simulink model "flatball_6dof-old"  (R2021b)
settings: Solver=ode1be  StartTime=0.0  StopTime=10  FixedStep=0.001  MaxStep=0.01  MinStep=0.01  RelTol=1e-3
values from neighbouring files (symbols this model uses):
  amb = evalin( 'base', 'amb')    [flatball_6dof_eqom.m]
  disc = evalin( 'base', 'disc')    [flatball_6dof_eqom.m]    (also in flatball_6dof_init.m = struct; flatball_init_disc_params.m = struct)
libraries: matrix_library x2, aerolibanim x1, simulink x1
(part 1 of 2)
settings Model: Creator=schae  LastModifiedBy=schae
settings SolverCC: InitialStep=0.01
settings DataIOCC: ReturnWorkspaceOutputsName=simout

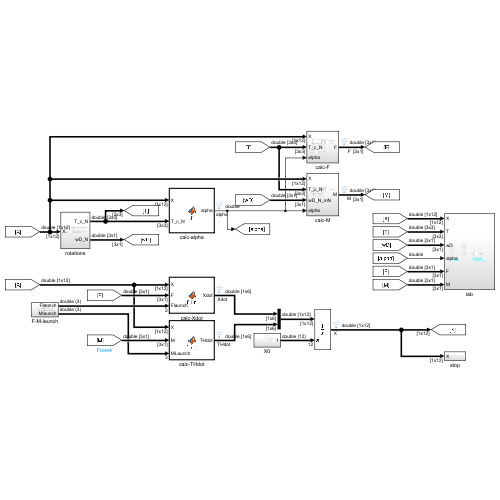
[thumbnail: Simulink's stored preview of the top-level diagram]
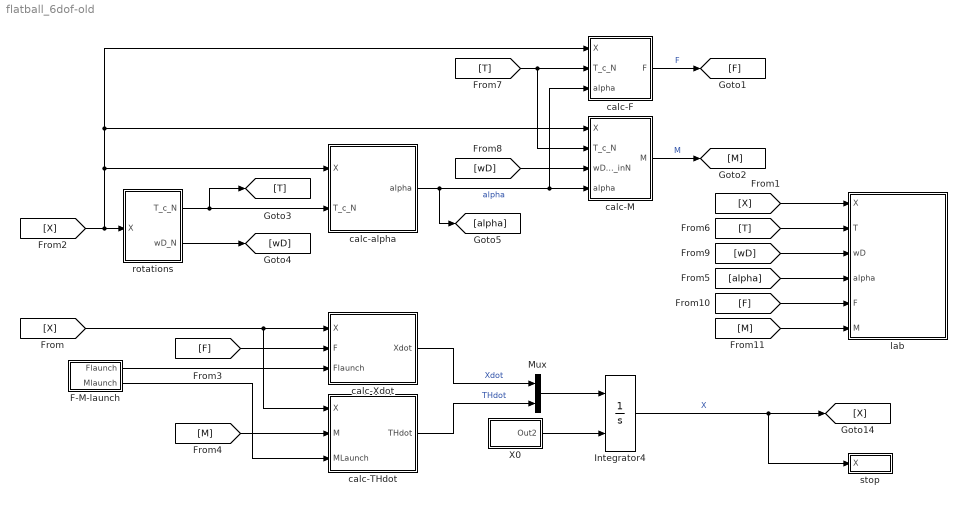
== system flatball_6dof-old ==
  F-M-launch : Subsystem
  Integrator4 : Integrator  InitialConditionSource=external
  Mux : Mux  Inputs=2
  X0 : Subsystem
  calc-F : Subsystem
  calc-M : Subsystem
  calc-THdot : MATLAB Function  TreatAsAtomicUnit=on
  calc-Xdot : MATLAB Function  TreatAsAtomicUnit=on
  calc-alpha : MATLAB Function  TreatAsAtomicUnit=on
  lab : Subsystem
  rotations : Subsystem
  stop : Subsystem
  wires:
  calc-Xdot/1(Xdot) -> Mux/1  "Xdot"
  X0/1(Out2) -> Integrator4/2
  Integrator4/1 -> stop/1(X), [X]  "X"
  [X] -> calc-THdot/1(X), calc-Xdot/1(X)
  calc-THdot/1(THdot) -> Mux/2  "THdot"
  Mux/1 -> Integrator4/1
  [wD] -> calc-M/3(wD_N_inN)
  calc-alpha/1(alpha) -> [alpha], calc-F/3(alpha), calc-M/4(alpha)  "alpha"
  rotations/1(T_c_N) -> [T], calc-alpha/2(T_c_N)
  rotations/2(wD_N) -> [wD]
  calc-F/1(F) -> [F]  "F"
  calc-M/1(M) -> [M]  "M"
  [T] -> calc-M/2(T_c_N), calc-F/2(T_c_N)
  [X] -> calc-F/1(X), calc-M/1(X), calc-alpha/1(X), rotations/1(X)
  [X] -> lab/1(X)
  [M] -> calc-THdot/2(M)
  [F] -> calc-Xdot/2(F)
  [T] -> lab/2(T)
  [wD] -> lab/3(wD)
  [F] -> lab/5(F)
  [M] -> lab/6(M)
  [alpha] -> lab/4(alpha)
  F-M-launch/1(Flaunch) -> calc-Xdot/3(Flaunch)
  F-M-launch/2(Mlaunch) -> calc-THdot/3(MLaunch)

== system flatball_6dof-old/F-M-launch ==
  Scope : Scope  NumInputPorts=2
  Subsystem : Subsystem
  Subsystem1 : Subsystem
  X0_hummel_f2302 : Constant  Commented=on  Value=[-0.90 -0.63 -0.91 13.42 -0.41 0.001 -0.07 0.21 5.03 -14.94 -1.48 54.25]
  Flaunch : Outport
  Mlaunch : Outport  Port=2
  wires:
  Subsystem1/1(Mlaunch) -> Scope/2, Mlaunch/1
  Subsystem/1(Flaunch) -> Scope/1, Flaunch/1

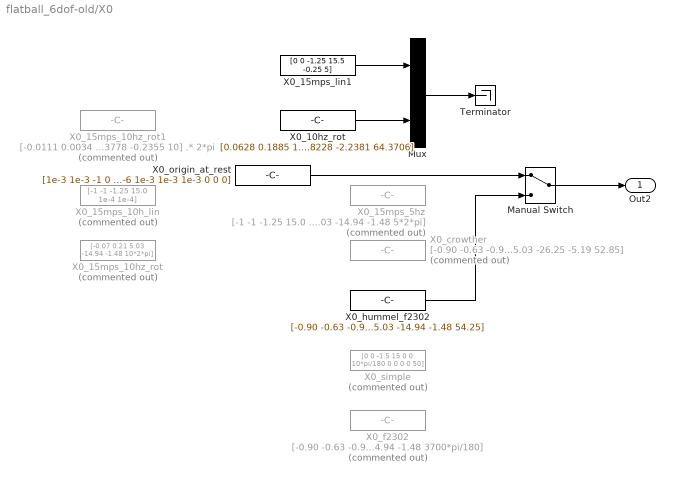
== system flatball_6dof-old/X0 ==
  Manual Switch : ManualSwitch
  Mux : Mux  Inputs=2
  Terminator : Terminator
  X0_10hz_rot : Constant  Value=[0.0628 0.1885 12.5664 1.8228 -2.2381 64.3706]
  X0_15mps_10h_lin : Constant  Commented=on  Value=[-1 -1 -1.25 15.0 1e-4 1e-4]
  X0_15mps_10hz_rot : Constant  Commented=on  Value=[-0.07 0.21 5.03 -14.94 -1.48 10*2*pi]
  X0_15mps_10hz_rot1 : Constant  Commented=on  Value=[-0.0111 0.0034 0.8005 -2.3778 -0.2355 10] .* 2*pi
  X0_15mps_5hz : Constant  Commented=on  Value=[-1 -1 -1.25 15.0 1e-4 1e-4 -0.07 0.21 5.03 -14.94 -1.48 5*2*pi]
  X0_15mps_lin1 : Constant  Value=[0 0 -1.25 15.5 -0.25 5]
  X0_crowther : Constant  Commented=on  Value=[-0.90 -0.63 -0.91 4.48 12.52 1.84 -0.07 0.21 5.03 -26.25 -5.19 52.85]
  X0_f2302 : Constant  Commented=on  Value=[-0.90 -0.63 -0.91 13.42 -0.41 0.001 -0.07 0.21 5.03 -14.94 -1.48 3700*pi/180]
  X0_hummel_f2302 : Constant  Value=[-0.90 -0.63 -0.91 13.42 -0.41 0.001 -0.07 0.21 5.03 -14.94 -1.48 54.25]
  X0_origin_at_rest : Constant  Value=[1e-3 1e-3 -1 0 0 -1e-6 1e-3 1e-3 1e-3 0 0 0]
  X0_simple : Constant  Commented=on  Value=[0 0 -1.5 15 0 0 10*pi/180 0 0 0 0 50]
  Out2 : Outport
  wires:
  Manual Switch/1 -> Out2/1
  X0_10hz_rot/1 -> Mux/2
  X0_15mps_lin1/1 -> Mux/1
  X0_hummel_f2302/1 -> Manual Switch/2
  Mux/1 -> Terminator/1
  X0_origin_at_rest/1 -> Manual Switch/1

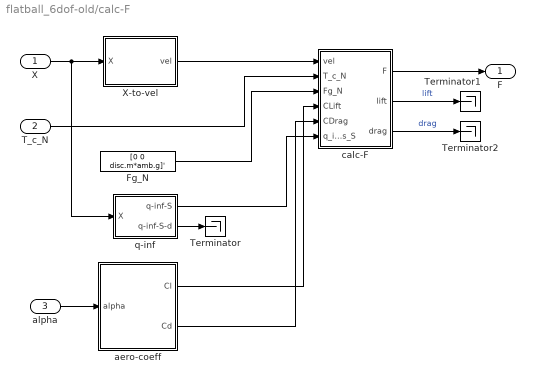
== system flatball_6dof-old/calc-F ==
  X : Inport
  T_c_N : Inport  Port=2
  alpha : Inport  Port=3
  Fg_N : Constant  Value=[0 0 disc.m*amb.g]'
  Terminator : Terminator
  Terminator1 : Terminator
  Terminator2 : Terminator
  X-to-vel : MATLAB Function  TreatAsAtomicUnit=on
  aero-coeff : Subsystem
  calc-F : MATLAB Function  TreatAsAtomicUnit=on
  q-inf : Subsystem
  F : Outport
  wires:
  X-to-vel/1(vel) -> calc-F/1(vel)
  X/1 -> q-inf/1(X), X-to-vel/1(X)
  T_c_N/1 -> calc-F/2(T_c_N)
  Fg_N/1 -> calc-F/3(Fg_N)
  calc-F/1(F) -> F/1
  q-inf/1(q-inf-S) -> calc-F/6(q_inf_times_S)
  alpha/1 -> aero-coeff/1(alpha)
  aero-coeff/1(Cl) -> calc-F/4(CLift)
  aero-coeff/2(Cd) -> calc-F/5(CDrag)
  q-inf/2(q-inf-S-d) -> Terminator/1
  calc-F/2(lift) -> Terminator1/1  "lift"
  calc-F/3(drag) -> Terminator2/1  "drag"

== system flatball_6dof-old/calc-M ==
  X : Inport
  T_c_N : Inport  Port=2
  wD_N_inN : Inport  Port=3
  alpha : Inport  Port=4
  Terminator : Terminator
  X-to-vel : MATLAB Function  TreatAsAtomicUnit=on
  aero-coeff : Subsystem
  calc-M : MATLAB Function  TreatAsAtomicUnit=on
  q-inf : Subsystem
  M : Outport
  wires:
  alpha/1 -> aero-coeff/1(alpha)
  calc-M/1(M) -> M/1
  T_c_N/1 -> calc-M/2(T_c_N)
  X/1 -> X-to-vel/1(X), q-inf/1(X)
  X-to-vel/1(vel) -> calc-M/1(vel)
  q-inf/2(q-inf-S-d) -> calc-M/5(q_inf_times_Sd)
  aero-coeff/1(Cm) -> calc-M/4(CMpitch)
  wD_N_inN/1 -> calc-M/3(wD_N_inN)
  q-inf/1(q-inf-S) -> Terminator/1

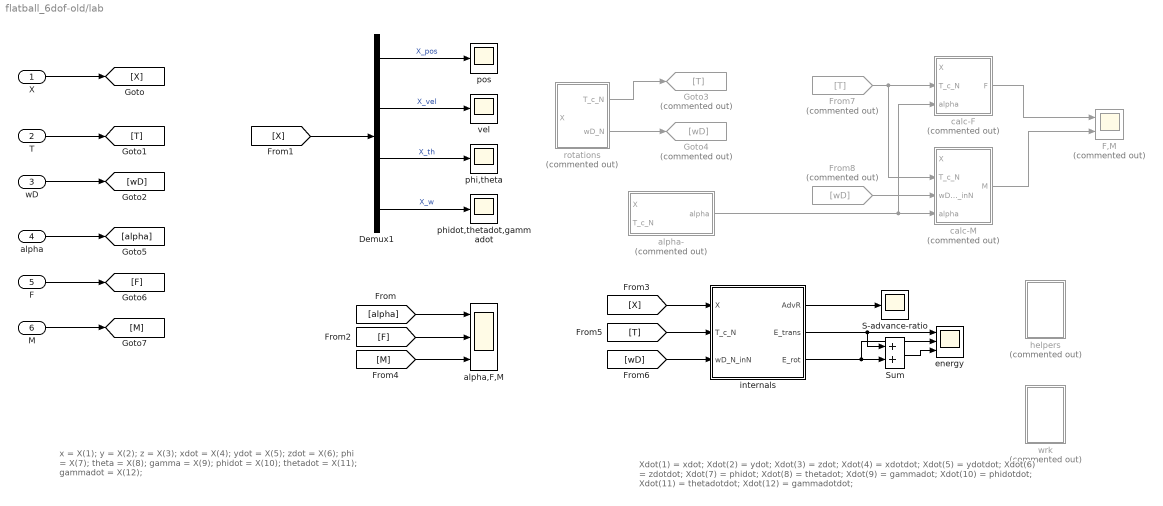
== system flatball_6dof-old/lab ==
  note: x = X(1); y = X(2); z = X(3);
      | xdot = X(4); ydot = X(5); zdot = X(6);
      |
      | phi = X(7); theta = X(8); gamma = X(9);
      | phidot = X(10); thetadot = X(11); gammadot = X(12);
  note: Xdot(1) = xdot; Xdot(2) = ydot; Xdot(3) = zdot;
      | Xdot(4) = xdotdot; Xdot(5) = ydotdot; Xdot(6) = zdotdot;
      |
      | Xdot(7) = phidot; Xdot(8) = thetadot; Xdot(9) = gammadot;
      | Xdot(10) = phidotdot; Xdot(11) = thetadotdot; Xdot(12) = gammadotdot;
  X : Inport
  T : Inport  Port=2
  wD : Inport  Port=3
  alpha : Inport  Port=4
  F : Inport  Port=5
  M : Inport  Port=6
  Demux1 : Demux  Outputs=[3 3 3 3]
  F,M : Scope  Commented=on  NumInputPorts=2
  From7 : From  Commented=on  GotoTag=T
  From8 : From  Commented=on  GotoTag=wD
  Goto3 : Goto  Commented=on  GotoTag=T
  Goto4 : Goto  Commented=on  GotoTag=wD
  S-advance-ratio : Scope
  Sum : Sum  Inputs=2
  alpha,F,M : Scope  NumInputPorts=3
  alpha- : MATLAB Function  Commented=on  TreatAsAtomicUnit=on
  calc-F : Subsystem  Commented=on
  calc-M : Subsystem  Commented=on
  energy : Scope  NumInputPorts=3
  helpers : Subsystem  Commented=on
  internals : MATLAB Function  TreatAsAtomicUnit=on
  phi,theta : Scope
  phidot,thetadot,gammadot : Scope
  pos : Scope
  rotations : Subsystem  Commented=on
  vel : Scope
  wrk : Subsystem  Commented=on
  wires:
  From7/1 -> calc-M/2(T_c_N), calc-F/2(T_c_N)
  alpha-/1(alpha) -> calc-F/3(alpha), calc-M/4(alpha)
  From8/1 -> calc-M/3(wD_N_inN)
  calc-M/1(M) -> F,M/2
  calc-F/1(F) -> F,M/1
  rotations/1(T_c_N) -> Goto3/1
  rotations/2(wD_N) -> Goto4/1
  internals/3(E_rot) -> Sum/2, energy/2
  [wD] -> internals/3(wD_N_inN)
  internals/1(AdvR) -> S-advance-ratio/1
  [T] -> internals/2(T_c_N)
  Sum/1 -> energy/3
  [X] -> internals/1(X)
  internals/2(E_trans) -> Sum/1, energy/1
  Demux1/4 -> phidot,thetadot,gammadot/1  "X_w"
  Demux1/3 -> phi,theta/1  "X_th"
  Demux1/1 -> pos/1  "X_pos"
  Demux1/2 -> vel/1  "X_vel"
  [X] -> Demux1/1
  X/1 -> [X]
  T/1 -> [T]
  wD/1 -> [wD]
  F/1 -> [F]
  alpha/1 -> [alpha]
  M/1 -> [M]
  [alpha] -> alpha,F,M/1
  [F] -> alpha,F,M/2
  [M] -> alpha,F,M/3

== system flatball_6dof-old/rotations ==
  X : Inport
  MatrixMultiply3 : Product  Multiplication=Matrix(*)
  Transpose : Math  Operator=transpose  SaturateOnIntegerOverflow=on
  Transpose1 : Math  Operator=transpose  SaturateOnIntegerOverflow=on
  X-to-T_c_N : MATLAB Function  TreatAsAtomicUnit=on
  X-to-wD_N_inC : MATLAB Function  TreatAsAtomicUnit=on
  T_c_N : Outport
  wD_N : Outport  Port=2
  wires:
  X-to-T_c_N/1(T_c_N) -> Transpose1/1, T_c_N/1
  Transpose1/1 -> MatrixMultiply3/1
  X-to-wD_N_inC/1(wD_N_inC) -> Transpose/1
  Transpose/1 -> MatrixMultiply3/2
  MatrixMultiply3/1 -> wD_N/1
  X/1 -> X-to-wD_N_inC/1(X), X-to-T_c_N/1(X)

== system flatball_6dof-old/stop ==
  X : Inport
  Compare To Constant : simulink/Logic and Bit Operations/Compare To Constant  relop=>=  const=0  OutDataTypeStr=boolean
  Selector : Selector  InputPortWidth=12  IndexOptions=Index vector (dialog)  Indices=[3]  OutputSizes=1
  Stop Simulation : Stop
  wires:
  Selector/1 -> Compare To Constant/1
  Compare To Constant/1 -> Stop Simulation/1
  X/1 -> Selector/1

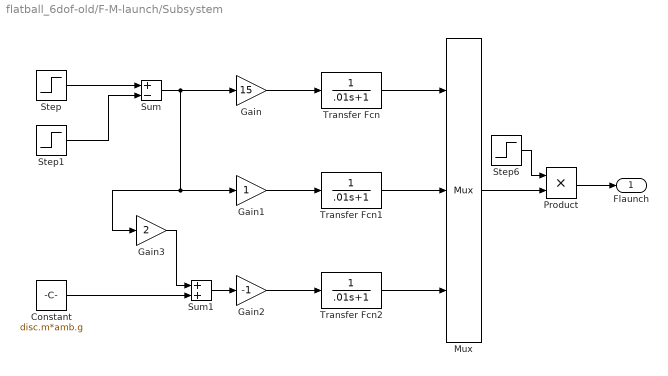
== system flatball_6dof-old/F-M-launch/Subsystem ==
  Constant : Constant  Value=disc.m*amb.g
  Gain : Gain  Gain=15
  Gain1 : Gain
  Gain2 : Gain  Gain=-1
  Gain3 : Gain  Gain=2
  Mux : Mux  Inputs=3
  Product : Product
  Step : Step  SampleTime=0
  Step1 : Step  Time=1.25  SampleTime=0
  Step6 : Step  Time=1.25  Before=1  After=0  SampleTime=0
  Sum : Sum  Inputs=+-
  Sum1 : Sum
  Transfer Fcn : TransferFcn  Denominator=[.01 1]
  Transfer Fcn1 : TransferFcn  Denominator=[.01 1]
  Transfer Fcn2 : TransferFcn  Denominator=[.01 1]
  Flaunch : Outport
  wires:
  Step1/1 -> Sum/2
  Step/1 -> Sum/1
  Sum/1 -> Gain/1, Gain3/1, Gain1/1
  Gain/1 -> Transfer Fcn/1
  Gain2/1 -> Transfer Fcn2/1
  Gain1/1 -> Transfer Fcn1/1
  Transfer Fcn/1 -> Mux/1
  Transfer Fcn1/1 -> Mux/2
  Transfer Fcn2/1 -> Mux/3
  Step6/1 -> Product/1
  Mux/1 -> Product/2
  Product/1 -> Flaunch/1
  Sum1/1 -> Gain2/1
  Constant/1 -> Sum1/2
  Gain3/1 -> Sum1/1

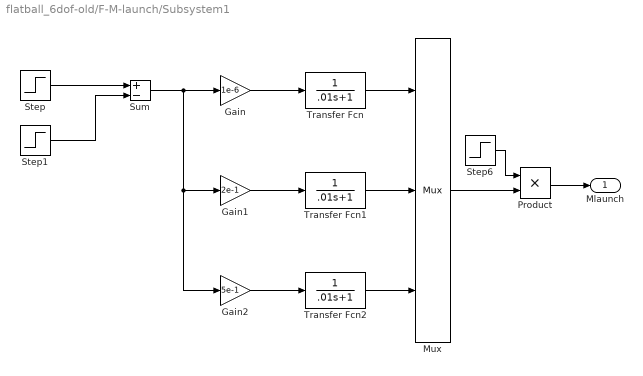
== system flatball_6dof-old/F-M-launch/Subsystem1 ==
  Gain : Gain  Gain=1e-6
  Gain1 : Gain  Gain=2e-1
  Gain2 : Gain  Gain=5e-1
  Mux : Mux  Inputs=3
  Product : Product
  Step : Step  SampleTime=0
  Step1 : Step  Time=1.25  SampleTime=0
  Step6 : Step  Time=3  Before=1  After=0  SampleTime=0
  Sum : Sum  Inputs=+-
  Transfer Fcn : TransferFcn  Denominator=[.01 1]
  Transfer Fcn1 : TransferFcn  Denominator=[.01 1]
  Transfer Fcn2 : TransferFcn  Denominator=[.01 1]
  Mlaunch : Outport
  wires:
  Gain1/1 -> Transfer Fcn1/1
  Gain2/1 -> Transfer Fcn2/1
  Gain/1 -> Transfer Fcn/1
  Sum/1 -> Gain1/1, Gain2/1, Gain/1
  Step/1 -> Sum/1
  Step1/1 -> Sum/2
  Transfer Fcn/1 -> Mux/1
  Transfer Fcn1/1 -> Mux/2
  Transfer Fcn2/1 -> Mux/3
  Mux/1 -> Product/2
  Step6/1 -> Product/1
  Product/1 -> Mlaunch/1

== system flatball_6dof-old/calc-F/aero-coeff ==
  alpha : Inport
  Subsystem : Subsystem
  Subsystem1 : Subsystem
  Cl : Outport
  Cd : Outport  Port=2
  wires:
  alpha/1 -> Subsystem1/1(alpha), Subsystem/1(alpha)
  Subsystem1/1(Cl) -> Cl/1
  Subsystem/1(Cd) -> Cd/1

== system flatball_6dof-old/calc-F/q-inf ==
  X : Inport
  Gain : Gain  Gain=0.5
  Product1 : Product  Inputs=3
  Product2 : Product
  S : Constant  Value=disc.A
  Square : Math  Operator=square  SaturateOnIntegerOverflow=on
  X-to-vel : MATLAB Function  TreatAsAtomicUnit=on
  d : Constant  Value=disc.d
  rho : Constant  Value=amb.rho
  vector-norm : MATLAB Function  TreatAsAtomicUnit=on
  q-inf-S : Outport
  q-inf-S-d : Outport  Port=2
  wires:
  Product1/1 -> Gain/1
  rho/1 -> Product1/3
  X/1 -> X-to-vel/1(X)
  vector-norm/1(norm) -> Square/1
  S/1 -> Product1/2
  Square/1 -> Product1/1
  Gain/1 -> Product2/1, q-inf-S/1
  X-to-vel/1(vel) -> vector-norm/1(vec)
  Product2/1 -> q-inf-S-d/1
  d/1 -> Product2/2

== system flatball_6dof-old/calc-M/aero-coeff ==
  alpha : Inport
  Subsystem2 : Subsystem
  Cm : Outport
  wires:
  alpha/1 -> Subsystem2/1(alpha)
  Subsystem2/1(Cm) -> Cm/1

== system flatball_6dof-old/calc-M/q-inf ==
  X : Inport
  Gain : Gain  Gain=0.5
  Product1 : Product  Inputs=3
  Product2 : Product
  S : Constant  Value=disc.A
  Square : Math  Operator=square  SaturateOnIntegerOverflow=on
  X-to-vel : MATLAB Function  TreatAsAtomicUnit=on
  d : Constant  Value=disc.d
  rho : Constant  Value=amb.rho
  vector-norm : MATLAB Function  TreatAsAtomicUnit=on
  q-inf-S : Outport
  q-inf-S-d : Outport  Port=2
  wires:
  d/1 -> Product2/2
  Product2/1 -> q-inf-S-d/1
  X-to-vel/1(vel) -> vector-norm/1(vec)
  Gain/1 -> q-inf-S/1, Product2/1
  Square/1 -> Product1/1
  S/1 -> Product1/2
  vector-norm/1(norm) -> Square/1
  X/1 -> X-to-vel/1(X)
  rho/1 -> Product1/3
  Product1/1 -> Gain/1

== system flatball_6dof-old/lab/calc-F ==
  X : Inport
  T_c_N : Inport  Port=2
  alpha : Inport  Port=3
  Fg_N : Constant  Value=[0 0 disc.m*amb.g]'
  Terminator : Terminator
  X-to-vel : MATLAB Function  TreatAsAtomicUnit=on
  aero-coeff : Subsystem
  calc-F : MATLAB Function  TreatAsAtomicUnit=on
  q-inf : Subsystem
  F : Outport
  wires:
  X-to-vel/1(vel) -> calc-F/1(vel)
  X/1 -> q-inf/1(X), X-to-vel/1(X)
  T_c_N/1 -> calc-F/2(T_c_N)
  Fg_N/1 -> calc-F/3(Fg_N)
  calc-F/1(F) -> F/1
  q-inf/1(q-inf-S) -> calc-F/6(q_inf_times_S)
  alpha/1 -> aero-coeff/1(alpha)
  aero-coeff/1(Cl) -> calc-F/4(CLift)
  aero-coeff/2(Cd) -> calc-F/5(CDrag)
  q-inf/2(q-inf-S-d) -> Terminator/1

== system flatball_6dof-old/lab/calc-M ==
  X : Inport
  T_c_N : Inport  Port=2
  wD_N_inN : Inport  Port=3
  alpha : Inport  Port=4
  Terminator : Terminator
  X-to-vel : MATLAB Function  TreatAsAtomicUnit=on
  aero-coeff : Subsystem
  calc-M : MATLAB Function  TreatAsAtomicUnit=on
  q-inf : Subsystem
  M : Outport
  wires:
  alpha/1 -> aero-coeff/1(alpha)
  calc-M/1(M) -> M/1
  T_c_N/1 -> calc-M/2(T_c_N)
  X/1 -> X-to-vel/1(X), q-inf/1(X)
  X-to-vel/1(vel) -> calc-M/1(vel)
  q-inf/2(q-inf-S-d) -> calc-M/5(q_inf_times_Sd)
  aero-coeff/1(Cm) -> calc-M/4(CMpitch)
  wD_N_inN/1 -> calc-M/3(wD_N_inN)
  q-inf/1(q-inf-S) -> Terminator/1

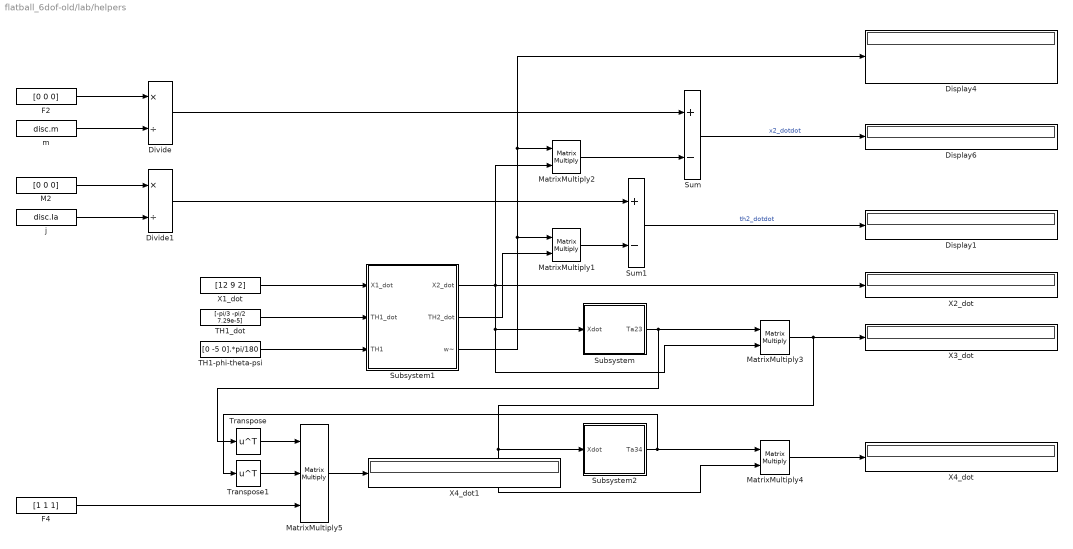
== system flatball_6dof-old/lab/helpers ==
  Display1 : Display
  Display4 : Display
  Display6 : Display
  Divide : Product  Inputs=*/
  Divide1 : Product  Inputs=*/
  F2 : Constant  Value=[0 0 0]
  F4 : Constant  Value=[1 1 1]
  M2 : Constant  Value=[0 0 0]
  MatrixMultiply{1..4} (4 alike) : Product  Multiplication=Matrix(*)
  MatrixMultiply5 : Product  Inputs=***  Multiplication=Matrix(*)
  Subsystem : Subsystem
  Subsystem1 : Subsystem
  Subsystem2 : Subsystem
  Sum : Sum  Inputs=+-
  Sum1 : Sum  Inputs=+-
  TH1-phi-theta-psi : Constant  Value=[0 -5 0].*pi/180
  TH1_dot : Constant  Value=[-pi/3 -pi/2 7.29e-5]
  Transpose : Math  Operator=transpose  SaturateOnIntegerOverflow=on
  Transpose1 : Math  Operator=transpose  SaturateOnIntegerOverflow=on
  X1_dot : Constant  Value=[12 9 2]
  X2_dot : Display
  X3_dot : Display
  X4_dot : Display
  X4_dot1 : Display
  j : Constant  Value=disc.Ia
  m : Constant  Value=disc.m
  wires:
  X1_dot/1 -> Subsystem1/1(X1_dot)
  TH1_dot/1 -> Subsystem1/2(TH1_dot)
  TH1-phi-theta-psi/1 -> Subsystem1/3(TH1)
  MatrixMultiply2/1 -> Sum/2
  Subsystem1/3(w~) -> MatrixMultiply1/1, Display4/1, MatrixMultiply2/1
  Subsystem1/1(X2_dot) -> MatrixMultiply2/2, X2_dot/1, MatrixMultiply3/2, Subsystem/1(Xdot)
  F2/1 -> Divide/1
  m/1 -> Divide/2
  Divide/1 -> Sum/1
  Sum/1 -> Display6/1  "x2_dotdot"
  j/1 -> Divide1/2
  M2/1 -> Divide1/1
  Divide1/1 -> Sum1/1
  MatrixMultiply1/1 -> Sum1/2
  Subsystem1/2(TH2_dot) -> MatrixMultiply1/2
  Sum1/1 -> Display1/1  "th2_dotdot"
  Subsystem/1(Ta23) -> Transpose/1, MatrixMultiply3/1
  MatrixMultiply3/1 -> MatrixMultiply4/2, Subsystem2/1(Xdot), X3_dot/1
  Subsystem2/1(Ta34) -> Transpose1/1, MatrixMultiply4/1
  MatrixMultiply4/1 -> X4_dot/1
  Transpose1/1 -> MatrixMultiply5/2
  Transpose/1 -> MatrixMultiply5/1
  F4/1 -> MatrixMultiply5/3
  MatrixMultiply5/1 -> X4_dot1/1

== system flatball_6dof-old/lab/rotations ==
  X : Inport
  MatrixMultiply3 : Product  Multiplication=Matrix(*)
  Transpose : Math  Operator=transpose  SaturateOnIntegerOverflow=on
  Transpose1 : Math  Operator=transpose  SaturateOnIntegerOverflow=on
  X-to-T_c_N : MATLAB Function  TreatAsAtomicUnit=on
  X-to-wD_N_inC : MATLAB Function  TreatAsAtomicUnit=on
  T_c_N : Outport
  wD_N : Outport  Port=2
  wires:
  X-to-T_c_N/1(T_c_N) -> Transpose1/1, T_c_N/1
  Transpose1/1 -> MatrixMultiply3/1
  X-to-wD_N_inC/1(wD_N_inC) -> Transpose/1
  Transpose/1 -> MatrixMultiply3/2
  MatrixMultiply3/1 -> wD_N/1
  X/1 -> X-to-wD_N_inC/1(X), X-to-T_c_N/1(X)

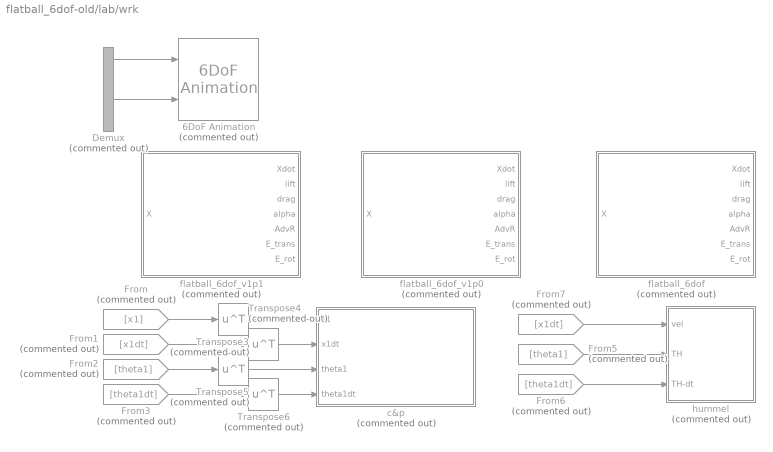
== system flatball_6dof-old/lab/wrk ==
  6DoF Animation : aerolibanim/6DoF Animation  Commented=on  u1=[-10 100 -20 100 -10 10]  u2=0.01  u3=5  u4=[1 0 -5]  u5=Fixed position  u6=[100 50 -500]  u7=10  u8=on
  Demux : Demux  Commented=on  Outputs=[3 3 3 3]
  From : From  Commented=on  GotoTag=x1
  From1 : From  Commented=on  GotoTag=x1dt
  From2 : From  Commented=on  GotoTag=theta1
  From3 : From  Commented=on  GotoTag=theta1dt
  From5 : From  Commented=on  GotoTag=theta1
  From6 : From  Commented=on  GotoTag=theta1dt
  From7 : From  Commented=on  GotoTag=x1dt
  Transpose{3..6} (4 alike) : Math  Commented=on  Operator=transpose  SaturateOnIntegerOverflow=on
  c&p : Subsystem  Commented=on
  flatball_6dof : MATLAB Function  Commented=on  TreatAsAtomicUnit=on
  flatball_6dof_v1p0 : MATLAB Function  Commented=on  TreatAsAtomicUnit=on
  flatball_6dof_v1p1 : MATLAB Function  Commented=on  TreatAsAtomicUnit=on
  hummel : Subsystem  Commented=on
  wires:
  From/1 -> Transpose3/1
  From2/1 -> Transpose5/1
  From3/1 -> Transpose6/1
  Demux/3 -> 6DoF Animation/2
  Transpose3/1 -> c&p/1(x1)
  Demux/1 -> 6DoF Animation/1
  From1/1 -> Transpose4/1
  Transpose5/1 -> c&p/3(theta1)
  Transpose4/1 -> c&p/2(x1dt)
  Transpose6/1 -> c&p/4(theta1dt)
  From5/1 -> hummel/2(TH)
  From6/1 -> hummel/3(TH-dt)
  From7/1 -> hummel/1(vel)

== system flatball_6dof-old/calc-F/aero-coeff/Subsystem ==
  alpha : Inport
  Cd0 : Constant  Value=disc.CD0
  Cda : Constant  Value=disc.CDa
  Product : Product
  Square : Math  Operator=square  SaturateOnIntegerOverflow=on
  Sum : Sum
  Sum1 : Sum
  alpha0 : Constant  Value=disc.alpha0
  Cd : Outport
  wires:
  Sum1/1 -> Cd/1
  Square/1 -> Product/2
  Product/1 -> Sum1/2
  Cda/1 -> Product/1
  Cd0/1 -> Sum1/1
  Sum/1 -> Square/1
  alpha0/1 -> Sum/2
  alpha/1 -> Sum/1

== system flatball_6dof-old/calc-F/aero-coeff/Subsystem1 ==
  alpha : Inport
  CL0 : Constant  Value=disc.CL0
  CLa : Constant  Value=disc.CLa
  Product : Product
  Sum1 : Sum
  Cl : Outport
  wires:
  alpha/1 -> Product/2
  CL0/1 -> Sum1/1
  CLa/1 -> Product/1
  Product/1 -> Sum1/2
  Sum1/1 -> Cl/1

== system flatball_6dof-old/calc-M/aero-coeff/Subsystem2 ==
  alpha : Inport
  CM0 : Constant  Value=disc.CM0
  CMa : Constant  Value=disc.CMa
  Product : Product
  Sum1 : Sum
  Cm : Outport
  wires:
  Sum1/1 -> Cm/1
  Product/1 -> Sum1/2
  CMa/1 -> Product/1
  CM0/1 -> Sum1/1
  alpha/1 -> Product/2

== system flatball_6dof-old/lab/calc-F/aero-coeff ==
  alpha : Inport
  Subsystem : Subsystem
  Subsystem1 : Subsystem
  Cl : Outport
  Cd : Outport  Port=2
  wires:
  alpha/1 -> Subsystem1/1(alpha), Subsystem/1(alpha)
  Subsystem1/1(Cl) -> Cl/1
  Subsystem/1(Cd) -> Cd/1

== system flatball_6dof-old/lab/calc-F/q-inf ==
  X : Inport
  Gain : Gain  Gain=0.5
  Product1 : Product  Inputs=3
  Product2 : Product
  S : Constant  Value=disc.A
  Square : Math  Operator=square  SaturateOnIntegerOverflow=on
  X-to-vel : MATLAB Function  TreatAsAtomicUnit=on
  d : Constant  Value=disc.d
  rho : Constant  Value=amb.rho
  vector-norm : MATLAB Function  TreatAsAtomicUnit=on
  q-inf-S : Outport
  q-inf-S-d : Outport  Port=2
  wires:
  Product1/1 -> Gain/1
  rho/1 -> Product1/3
  X/1 -> X-to-vel/1(X)
  vector-norm/1(norm) -> Square/1
  S/1 -> Product1/2
  Square/1 -> Product1/1
  Gain/1 -> Product2/1, q-inf-S/1
  X-to-vel/1(vel) -> vector-norm/1(vec)
  Product2/1 -> q-inf-S-d/1
  d/1 -> Product2/2

== system flatball_6dof-old/lab/calc-M/aero-coeff ==
  alpha : Inport
  Subsystem2 : Subsystem
  Cm : Outport
  wires:
  alpha/1 -> Subsystem2/1(alpha)
  Subsystem2/1(Cm) -> Cm/1

== system flatball_6dof-old/lab/calc-M/q-inf ==
  X : Inport
  Gain : Gain  Gain=0.5
  Product1 : Product  Inputs=3
  Product2 : Product
  S : Constant  Value=disc.A
  Square : Math  Operator=square  SaturateOnIntegerOverflow=on
  X-to-vel : MATLAB Function  TreatAsAtomicUnit=on
  d : Constant  Value=disc.d
  rho : Constant  Value=amb.rho
  vector-norm : MATLAB Function  TreatAsAtomicUnit=on
  q-inf-S : Outport
  q-inf-S-d : Outport  Port=2
  wires:
  d/1 -> Product2/2
  Product2/1 -> q-inf-S-d/1
  X-to-vel/1(vel) -> vector-norm/1(vec)
  Gain/1 -> q-inf-S/1, Product2/1
  Square/1 -> Product1/1
  S/1 -> Product1/2
  vector-norm/1(norm) -> Square/1
  X/1 -> X-to-vel/1(X)
  rho/1 -> Product1/3
  Product1/1 -> Gain/1

== system flatball_6dof-old/lab/helpers/Subsystem ==
  Xdot : Inport
  Display : Display
  Gain : Gain  Gain=-1
  Ground2 : Ground
  Ground3 : Ground
  Ta1 : MATLAB Function  TreatAsAtomicUnit=on
  zero-side-slip-angle : MATLAB Function  TreatAsAtomicUnit=on
  Ta23 : Outport
  wires:
  Ground2/1 -> Ta1/2(theta)
  Gain/1 -> Ta1/3(psi)
  Ground3/1 -> Ta1/1(phi)
  Ta1/1(T) -> Ta23/1  "Ta23"
  zero-side-slip-angle/1(beta) -> Display/1, Gain/1  "beta"
  Xdot/1 -> zero-side-slip-angle/1(Xdot)

== system flatball_6dof-old/lab/helpers/Subsystem1 ==
  X1_dot : Inport
  TH1_dot : Inport  Port=2
  TH1 : Inport  Port=3
  Display : Display
  Display1 : Display
  MatrixMultiply : Product  Multiplication=Matrix(*)
  MatrixMultiply1 : Product  Multiplication=Matrix(*)
  transformation-matrices : Subsystem
  w_ : MATLAB Function  TreatAsAtomicUnit=on
  X2_dot : Outport
  TH2_dot : Outport  Port=2
  w~ : Outport  Port=3
  wires:
  MatrixMultiply/1 -> Display/1, X2_dot/1
  MatrixMultiply1/1 -> w_/1(THdot), Display1/1, TH2_dot/1
  transformation-matrices/1(Ta12) -> MatrixMultiply/1
  transformation-matrices/2(Tr12) -> MatrixMultiply1/1
  X1_dot/1 -> MatrixMultiply/2
  TH1_dot/1 -> MatrixMultiply1/2
  TH1/1 -> transformation-matrices/1(TH)
  w_/1(M) -> w~/1  "w_"

== system flatball_6dof-old/lab/helpers/Subsystem2 ==
  Xdot : Inport
  Display : Display
  Ground : Ground
  Ground1 : Ground
  Ta2 : MATLAB Function  TreatAsAtomicUnit=on
  angle-of-attack : MATLAB Function  TreatAsAtomicUnit=on
  Ta34 : Outport
  wires:
  Ground1/1 -> Ta2/3(psi)
  Ta2/1(T) -> Ta34/1  "Ta34"
  angle-of-attack/1(alpha) -> Display/1, Ta2/2(theta)  "alpha"
  Xdot/1 -> angle-of-attack/1(Xdot)
  Ground/1 -> Ta2/1(phi)

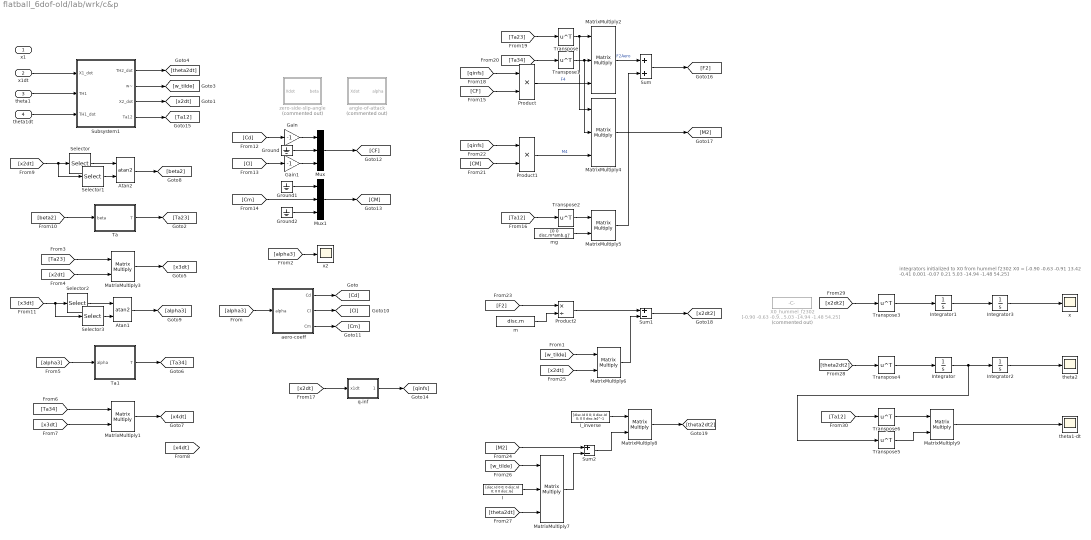
== system flatball_6dof-old/lab/wrk/c&p ==
  note: integrators initialized to X0 from hummel f2302
      | X0 = [-0.90 -0.63 -0.91 13.42 -0.41 0.001 -0.07 0.21 5.03 -14.94 -1.48 54.25]
  x1 : Inport
  x1dt : Inport  Port=2
  theta1 : Inport  Port=3
  theta1dt : Inport  Port=4
  Atan1 : Trigonometry  Operator=atan2
  Atan2 : Trigonometry  Operator=atan2
  Gain : Gain  Gain=-1
  Gain1 : Gain  Gain=-1
  Ground : Ground
  Ground1 : Ground
  Ground2 : Ground
  I : Constant  Value=[disc.Id 0 0; 0 disc.Id 0; 0 0 disc.Ia]
  I_inverse : Constant  Value=[disc.Id 0 0; 0 disc.Id 0; 0 0 disc.Ia]^-1
  Integrator : Integrator  InitialCondition=[-14.94 -1.48 54.25]
  Integrator1 : Integrator  InitialCondition=[13.42 -0.41 0.001]
  Integrator2 : Integrator  InitialCondition=[-0.07 0.21 5.03]
  Integrator3 : Integrator  InitialCondition=[-0.90 -0.63 -0.91]
  MatrixMultiply{1,3,5..6,8..9} (6 alike) : Product  Multiplication=Matrix(*)
  MatrixMultiply2 : Product  Inputs=3  Multiplication=Matrix(*)
  MatrixMultiply4 : Product  Inputs=3  Multiplication=Matrix(*)
  MatrixMultiply7 : Product  Inputs=3  Multiplication=Matrix(*)
  Mux : Mux  Inputs=3
  Mux1 : Mux  Inputs=3
  Product : Product
  Product1 : Product
  Product2 : Product  Inputs=*/
  Selector : Selector  InputPortWidth=3  IndexOptions=Index vector (dialog)  Indices=[2]  OutputSizes=1
  Selector1 : Selector  InputPortWidth=3  IndexOptions=Index vector (dialog)  Indices=[1]  OutputSizes=1
  Selector2 : Selector  InputPortWidth=3  IndexOptions=Index vector (dialog)  Indices=[3]  OutputSizes=1
  Selector3 : Selector  InputPortWidth=3  IndexOptions=Index vector (dialog)  Indices=[1]  OutputSizes=1
  Subsystem1 : Subsystem
  Sum : Sum
  Sum1 : Sum  Inputs=+-
  Sum2 : Sum  Inputs=+-
  Ta : MATLAB Function  TreatAsAtomicUnit=on
  Ta1 : MATLAB Function  TreatAsAtomicUnit=on
  Transpose{,1..6} (7 alike) : Math  Operator=transpose  SaturateOnIntegerOverflow=on
  X0_hummel_f2302 : Constant  Commented=on  Value=[-0.90 -0.63 -0.91 13.42 -0.41 0.001 -0.07 0.21 5.03 -14.94 -1.48 54.25]
  aero-coeff : Subsystem
  angle-of-attack : MATLAB Function  Commented=on  TreatAsAtomicUnit=on
  m : Constant  Value=disc.m
  mg : Constant  Value=[0 0 disc.m*amb.g]'
  q-inf : Subsystem
  theta1-dt : Scope
  theta2 : Scope
  x : Scope
  x2 : Scope
  zero-side-slip-angle : MATLAB Function  Commented=on  TreatAsAtomicUnit=on
  wires:
  x1dt/1 -> Subsystem1/1(X1_dot)
  theta1dt/1 -> Subsystem1/3(TH1_dot)
  theta1/1 -> Subsystem1/2(TH1)
  Ta/1(T) -> [Ta23]
  Subsystem1/2(w~) -> [w_tilde]
  Subsystem1/1(TH2_dot) -> [theta2dt]
  [beta2] -> Ta/1(beta)
  MatrixMultiply3/1 -> [x3dt]
  [alpha3] -> Ta1/1(alpha)
  Ta1/1(T) -> [Ta34]
  MatrixMultiply1/1 -> [x4dt]
  [x2dt] -> Selector1/1, Selector/1
  Atan2/1 -> [beta2]
  Atan1/1 -> [alpha3]
  aero-coeff/1(Cd) -> [Cd]
  aero-coeff/3(Cm) -> [Cm]
  aero-coeff/2(Cl) -> [Cl]
  [alpha3] -> aero-coeff/1(alpha)
  [Cd] -> Gain/1
  [Cl] -> Gain1/1
  Ground/1 -> Mux/2
  Mux/1 -> [CF]
  Gain/1 -> Mux/1
  Gain1/1 -> Mux/3
  [Cm] -> Mux1/2
  Ground1/1 -> Mux1/1
  Ground2/1 -> Mux1/3
  Mux1/1 -> [CM]
  [x2dt] -> q-inf/1(x1dt)
  q-inf/1(q-inf-S) -> [qinfs]
  [qinfs] -> Product/1
  [CF] -> Product/2
  [Ta34] -> Transpose1/1
  [Ta23] -> Transpose/1
  Transpose/1 -> MatrixMultiply4/1, MatrixMultiply2/1
  Transpose1/1 -> MatrixMultiply4/2, MatrixMultiply2/2
  Product/1 -> MatrixMultiply2/3  "F4"
  [CM] -> Product1/2
  [qinfs] -> Product1/1
  Product1/1 -> MatrixMultiply4/3  "M4"
  [Ta23] -> MatrixMultiply3/1
  [x2dt] -> MatrixMultiply3/2
  [x3dt] -> MatrixMultiply1/2
  [Ta34] -> MatrixMultiply1/1
  Subsystem1/4(Ta12) -> [Ta12]
  [Ta12] -> Transpose2/1
  Transpose2/1 -> MatrixMultiply5/1
  mg/1 -> MatrixMultiply5/2
  MatrixMultiply2/1 -> Sum/1  "F2Aero"
  MatrixMultiply5/1 -> Sum/2
  Sum/1 -> [F2]
  MatrixMultiply4/1 -> [M2]
  [F2] -> Product2/1
  m/1 -> Product2/2
  Product2/1 -> Sum1/1
  [w_tilde] -> MatrixMultiply6/1
  [x2dt] -> MatrixMultiply6/2
  MatrixMultiply6/1 -> Sum1/2
  Sum1/1 -> [x2dt2]
  [M2] -> Sum2/1
  [theta2dt] -> MatrixMultiply7/3
  [w_tilde] -> MatrixMultiply7/1
  I/1 -> MatrixMultiply7/2
  MatrixMultiply7/1 -> Sum2/2
  MatrixMultiply8/1 -> [theta2dt2]
  [theta2dt2] -> Transpose4/1
  [x2dt2] -> Transpose3/1
  Integrator/1 -> Integrator2/1, Transpose5/1
  Integrator1/1 -> Integrator3/1
  Integrator2/1 -> theta2/1
  Integrator3/1 -> x/1
  I_inverse/1 -> MatrixMultiply8/1
  Sum2/1 -> MatrixMultiply8/2
  Subsystem1/3(X2_dot) -> [x2dt]
  Transpose3/1 -> Integrator1/1
  Transpose4/1 -> Integrator/1
  [alpha3] -> x2/1
  Selector/1 -> Atan2/1
  Selector1/1 -> Atan2/2
  Selector3/1 -> Atan1/2
  Selector2/1 -> Atan1/1
  [x3dt] -> Selector3/1, Selector2/1
  Transpose5/1 -> MatrixMultiply9/2
  [Ta12] -> Transpose6/1
  Transpose6/1 -> MatrixMultiply9/1
  MatrixMultiply9/1 -> theta1-dt/1

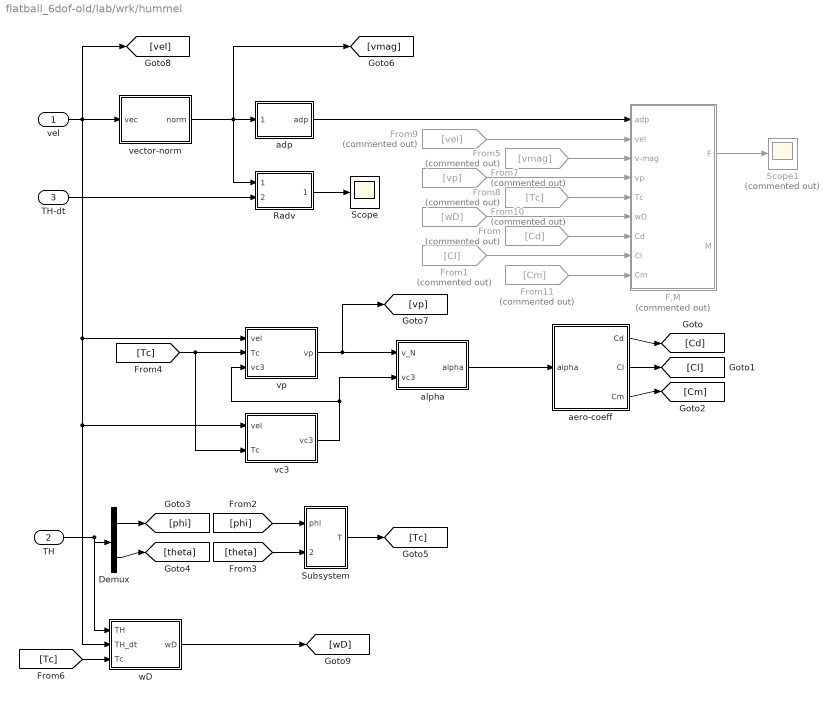
== system flatball_6dof-old/lab/wrk/hummel ==
  vel : Inport
  TH : Inport  Port=2
  TH-dt : Inport  Port=3
  Demux : Demux  Outputs=2
  F,M : Subsystem  Commented=on
  From : From  Commented=on  GotoTag=Cd
  From1 : From  Commented=on  GotoTag=Cl
  From10 : From  Commented=on  GotoTag=wD
  From11 : From  Commented=on  GotoTag=Cm
  From5 : From  Commented=on  GotoTag=vmag
  From7 : From  Commented=on  GotoTag=vp
  From8 : From  Commented=on  GotoTag=Tc
  From9 : From  Commented=on  GotoTag=vel
  Radv : Subsystem
  Scope : Scope
  Scope1 : Scope  Commented=on
  Subsystem : Subsystem
  adp : Subsystem
  aero-coeff : Subsystem
  alpha : MATLAB Function  TreatAsAtomicUnit=on
  vc3 : MATLAB Function  TreatAsAtomicUnit=on
  vector-norm : MATLAB Function  TreatAsAtomicUnit=on
  vp : MATLAB Function  TreatAsAtomicUnit=on
  wD : MATLAB Function  TreatAsAtomicUnit=on
  wires:
  aero-coeff/1(Cd) -> [Cd]
  aero-coeff/2(Cl) -> [Cl]
  aero-coeff/3(Cm) -> [Cm]
  adp/1(adp) -> F,M/1(adp)
  vel/1 -> [vel], wD/2(TH_dt), vc3/1(vel), vp/1(vel), vector-norm/1(vec)
  TH/1 -> wD/1(TH), Demux/1
  Demux/2 -> [theta]
  Demux/1 -> [phi]
  [phi] -> Subsystem/1(phi)
  [theta] -> Subsystem/2(theta)
  vector-norm/1(norm) -> Radv/1(v-mag), [vmag], adp/1(v-mag)
  Subsystem/1(T) -> [Tc]
  vp/1(vp) -> [vp], alpha/1(v_N)
  [Tc] -> vc3/2(Tc), vp/2(Tc)
  vc3/1(vc3) -> vp/3(vc3), alpha/2(vc3)
  alpha/1(alpha) -> aero-coeff/1(alpha)
  TH-dt/1 -> Radv/2(TH-dt)
  Radv/1(Radv) -> Scope/1
  [Tc] -> wD/3(Tc)
  wD/1(wD) -> [wD]
  From5/1 -> F,M/3(v-mag)
  From7/1 -> F,M/4(vp)
  From8/1 -> F,M/5(Tc)
  F,M/1(F) -> Scope1/1
  From9/1 -> F,M/2(vel)
  From10/1 -> F,M/6(wD)
  From/1 -> F,M/7(Cd)
  From1/1 -> F,M/8(Cl)
  From11/1 -> F,M/9(Cm)

== system flatball_6dof-old/lab/calc-F/aero-coeff/Subsystem ==
  alpha : Inport
  Cd0 : Constant  Value=disc.CD0
  Cda : Constant  Value=disc.CDa
  Product : Product
  Square : Math  Operator=square  SaturateOnIntegerOverflow=on
  Sum : Sum
  Sum1 : Sum
  alpha0 : Constant  Value=disc.alpha0
  Cd : Outport
  wires:
  Sum1/1 -> Cd/1
  Square/1 -> Product/2
  Product/1 -> Sum1/2
  Cda/1 -> Product/1
  Cd0/1 -> Sum1/1
  Sum/1 -> Square/1
  alpha0/1 -> Sum/2
  alpha/1 -> Sum/1

== system flatball_6dof-old/lab/calc-F/aero-coeff/Subsystem1 ==
  alpha : Inport
  CL0 : Constant  Value=disc.CL0
  CLa : Constant  Value=disc.CLa
  Product : Product
  Sum1 : Sum
  Cl : Outport
  wires:
  alpha/1 -> Product/2
  CL0/1 -> Sum1/1
  CLa/1 -> Product/1
  Product/1 -> Sum1/2
  Sum1/1 -> Cl/1

== system flatball_6dof-old/lab/calc-M/aero-coeff/Subsystem2 ==
  alpha : Inport
  CM0 : Constant  Value=disc.CM0
  CMa : Constant  Value=disc.CMa
  Product : Product
  Sum1 : Sum
  Cm : Outport
  wires:
  Sum1/1 -> Cm/1
  Product/1 -> Sum1/2
  CMa/1 -> Product/1
  CM0/1 -> Sum1/1
  alpha/1 -> Product/2

== system flatball_6dof-old/lab/helpers/Subsystem1/transformation-matrices ==
  TH : Inport
  Ta : MATLAB Function  TreatAsAtomicUnit=on
  Tr : MATLAB Function  TreatAsAtomicUnit=on
  Ta12 : Outport
  Tr12 : Outport  Port=2
  wires:
  TH/1 -> Ta/1(TH), Tr/1(TH)
  Ta/1(M) -> Ta12/1  "Ta12"
  Tr/1(M) -> Tr12/1  "Tr12"

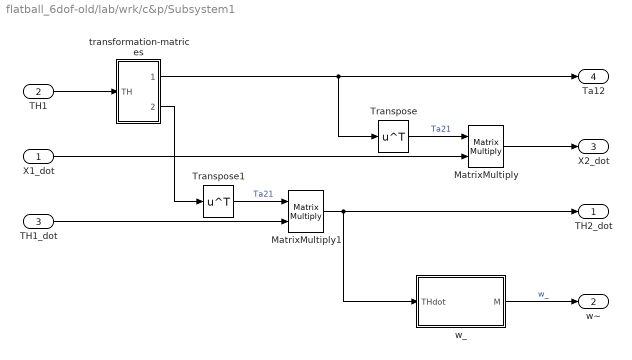
== system flatball_6dof-old/lab/wrk/c&p/Subsystem1 ==
  X1_dot : Inport
  TH1 : Inport  Port=2
  TH1_dot : Inport  Port=3
  MatrixMultiply : Product  Multiplication=Matrix(*)
  MatrixMultiply1 : Product  Multiplication=Matrix(*)
  Transpose : Math  Operator=transpose  SaturateOnIntegerOverflow=on
  Transpose1 : Math  Operator=transpose  SaturateOnIntegerOverflow=on
  transformation-matrices : Subsystem
  w_ : MATLAB Function  TreatAsAtomicUnit=on
  TH2_dot : Outport
  w~ : Outport  Port=2
  X2_dot : Outport  Port=3
  Ta12 : Outport  Port=4
  wires:
  MatrixMultiply/1 -> X2_dot/1
  MatrixMultiply1/1 -> w_/1(THdot), TH2_dot/1
  transformation-matrices/1(Ta12) -> Transpose/1, Ta12/1
  transformation-matrices/2(Tr12) -> Transpose1/1
  X1_dot/1 -> MatrixMultiply/2
  TH1_dot/1 -> MatrixMultiply1/2
  TH1/1 -> transformation-matrices/1(TH)
  w_/1(M) -> w~/1  "w_"
  Transpose/1 -> MatrixMultiply/1  "Ta21"
  Transpose1/1 -> MatrixMultiply1/1  "Ta21"

== system flatball_6dof-old/lab/wrk/c&p/aero-coeff ==
  alpha : Inport
  Subsystem : Subsystem
  Subsystem1 : Subsystem
  Subsystem2 : Subsystem
  Cd : Outport
  Cl : Outport  Port=2
  Cm : Outport  Port=3
  wires:
  alpha/1 -> Subsystem2/1(alpha), Subsystem1/1(alpha), Subsystem/1(alpha)
  Subsystem2/1(Cm) -> Cm/1
  Subsystem1/1(Cl) -> Cl/1
  Subsystem/1(Cd) -> Cd/1

== system flatball_6dof-old/lab/wrk/c&p/q-inf ==
  x1dt : Inport
  Gain : Gain  Gain=0.5
  Product1 : Product  Inputs=3
  S : Constant  Value=disc.A
  Square : Math  Operator=square  SaturateOnIntegerOverflow=on
  rho : Constant  Value=amb.rho
  vector-norm : MATLAB Function  TreatAsAtomicUnit=on
  q-inf-S : Outport
  wires:
  Product1/1 -> Gain/1
  rho/1 -> Product1/3
  x1dt/1 -> vector-norm/1(vec)
  vector-norm/1(norm) -> Square/1
  S/1 -> Product1/2
  Square/1 -> Product1/1
  Gain/1 -> q-inf-S/1

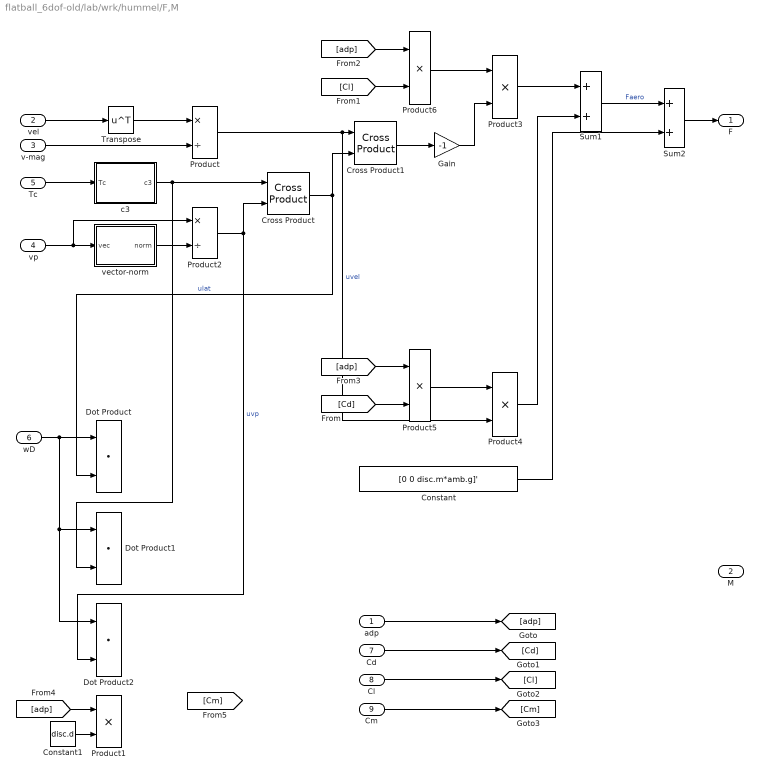
== system flatball_6dof-old/lab/wrk/hummel/F,M ==
  adp : Inport
  vel : Inport  Port=2
  v-mag : Inport  Port=3
  vp : Inport  Port=4
  Tc : Inport  Port=5
  wD : Inport  Port=6
  Cd : Inport  Port=7
  Cl : Inport  Port=8
  Cm : Inport  Port=9
  Constant : Constant  Value=[0 0 disc.m*amb.g]'
  Constant1 : Constant  Value=disc.d
  Cross Product : matrix_library/Cross Product
      settings: SourceProductBaseCode=SL
  Cross Product1 : matrix_library/Cross Product
      settings: SourceProductBaseCode=SL
  Dot Product : DotProduct  InputSameDT=on  OutDataTypeStr=Inherit: Inherit via internal rule
  Dot Product1 : DotProduct  InputSameDT=on  OutDataTypeStr=Inherit: Inherit via internal rule
  Dot Product2 : DotProduct  InputSameDT=on  OutDataTypeStr=Inherit: Inherit via internal rule
  Gain : Gain  Gain=-1
  Product : Product  Inputs=*/
  Product1 : Product  Inputs=**
  Product2 : Product  Inputs=*/
  Product{3..6} (4 alike) : Product
  Sum1 : Sum
  Sum2 : Sum
  Transpose : Math  Operator=transpose  SaturateOnIntegerOverflow=on
  c3 : MATLAB Function  TreatAsAtomicUnit=on
  vector-norm : MATLAB Function  TreatAsAtomicUnit=on
  F : Outport
  M : Outport  Port=2
  wires:
  vel/1 -> Transpose/1
  v-mag/1 -> Product/2
  vp/1 -> Product2/1, vector-norm/1(vec)
  vector-norm/1(norm) -> Product2/2
  Product2/1 -> Dot Product2/2, Cross Product/2  "uvp"
  Tc/1 -> c3/1(Tc)
  c3/1(c3) -> Dot Product1/2, Cross Product/1
  Cross Product/1 -> Cross Product1/2, Dot Product/2  "ulat"
  Product/1 -> Cross Product1/1, Product4/2  "uvel"
  Cross Product1/1 -> Gain/1
  Gain/1 -> Product3/2
  Product3/1 -> Sum1/1
  Product4/1 -> Sum1/2
  Sum1/1 -> Sum2/1  "Faero"
  Transpose/1 -> Product/1
  Sum2/1 -> F/1
  Constant/1 -> Sum2/2
  adp/1 -> [adp]
  Constant1/1 -> Product1/2
  wD/1 -> Dot Product2/1, Dot Product1/1, Dot Product/1
  Product5/1 -> Product4/1
  [Cl] -> Product6/2
  [Cd] -> Product5/2
  Product6/1 -> Product3/1
  [adp] -> Product6/1
  [adp] -> Product5/1
  Cd/1 -> [Cd]
  Cl/1 -> [Cl]
  Cm/1 -> [Cm]
  [adp] -> Product1/1

== system flatball_6dof-old/lab/wrk/hummel/Radv ==
  v-mag : Inport
  TH-dt : Inport  Port=2
  Gain : Gain  Gain=0.5
  Product1 : Product  Inputs=**/
  Selector : Selector  InputPortWidth=3  IndexOptions=Index vector (dialog)  Indices=[3]  OutputSizes=1
  "[0.5 .. inf]" : Saturate  UpperLimit=inf  LowerLimit=0.50
  d : Constant  Value=disc.d
  Radv : Outport
  wires:
  Product1/1 -> Radv/1
  d/1 -> Gain/1
  TH-dt/1 -> Selector/1
  Selector/1 -> Product1/1
  Gain/1 -> Product1/2
  v-mag/1 -> "[0.5 .. inf]"/1
  "[0.5 .. inf]"/1 -> Product1/3

== system flatball_6dof-old/lab/wrk/hummel/Subsystem ==
  phi : Inport
  theta : Inport  Port=2
  Tc : MATLAB Function  TreatAsAtomicUnit=on
  T : Outport
  wires:
  theta/1 -> Tc/2(theta)
  phi/1 -> Tc/1(phi)
  Tc/1(Tc) -> T/1

== system flatball_6dof-old/lab/wrk/hummel/adp ==
  v-mag : Inport
  A : Constant  Value=disc.A
  Gain : Gain  Gain=0.5
  Product : Product
  Product1 : Product  Inputs=3
  rho : Constant  Value=amb.rho
  adp : Outport
  wires:
  Product1/1 -> adp/1
  rho/1 -> Product/1
  A/1 -> Product/2
  Product/1 -> Gain/1
  v-mag/1 -> Product1/2, Product1/1
  Gain/1 -> Product1/3

== system flatball_6dof-old/lab/wrk/hummel/aero-coeff ==
  alpha : Inport
  Subsystem : Subsystem
  Subsystem1 : Subsystem
  Subsystem2 : Subsystem
  Cd : Outport
  Cl : Outport  Port=2
  Cm : Outport  Port=3
  wires:
  alpha/1 -> Subsystem2/1(alpha), Subsystem1/1(alpha), Subsystem/1(alpha)
  Subsystem2/1(Cm) -> Cm/1
  Subsystem1/1(Cl) -> Cl/1
  Subsystem/1(Cd) -> Cd/1

== system flatball_6dof-old/lab/wrk/c&p/Subsystem1/transformation-matrices ==
  TH : Inport
  Ta : MATLAB Function  TreatAsAtomicUnit=on
  Tr : MATLAB Function  TreatAsAtomicUnit=on
  Ta12 : Outport
  Tr12 : Outport  Port=2
  wires:
  TH/1 -> Ta/1(TH), Tr/1(TH)
  Ta/1(Ta12) -> Ta12/1
  Tr/1(Tr12) -> Tr12/1

== system flatball_6dof-old/lab/wrk/c&p/aero-coeff/Subsystem ==
  alpha : Inport
  Cd0 : Constant  Value=disc.CD0
  Cda : Constant  Value=disc.CDa
  Product : Product
  Square : Math  Operator=square  SaturateOnIntegerOverflow=on
  Sum : Sum
  Sum1 : Sum
  alpha0 : Constant  Value=disc.alpha0
  Cd : Outport
  wires:
  Sum1/1 -> Cd/1
  Square/1 -> Product/2
  Product/1 -> Sum1/2
  Cda/1 -> Product/1
  Cd0/1 -> Sum1/1
  Sum/1 -> Square/1
  alpha0/1 -> Sum/2
  alpha/1 -> Sum/1

== system flatball_6dof-old/lab/wrk/c&p/aero-coeff/Subsystem1 ==
  alpha : Inport
  CL0 : Constant  Value=disc.CL0
  CLa : Constant  Value=disc.CLa
  Product : Product
  Sum1 : Sum
  Cl : Outport
  wires:
  alpha/1 -> Product/2
  CL0/1 -> Sum1/1
  CLa/1 -> Product/1
  Product/1 -> Sum1/2
  Sum1/1 -> Cl/1

== system flatball_6dof-old/lab/wrk/c&p/aero-coeff/Subsystem2 ==
  alpha : Inport
  CM0 : Constant  Value=disc.CM0
  CMa : Constant  Value=disc.CMa
  Product : Product
  Sum1 : Sum
  Cm : Outport
  wires:
  Sum1/1 -> Cm/1
  Product/1 -> Sum1/2
  CMa/1 -> Product/1
  CM0/1 -> Sum1/1
  alpha/1 -> Product/2

== system flatball_6dof-old/lab/wrk/hummel/aero-coeff/Subsystem ==
  alpha : Inport
  Cd0 : Constant  Value=disc.CD0
  Cda : Constant  Value=disc.CDa
  Product : Product
  Square : Math  Operator=square  SaturateOnIntegerOverflow=on
  Sum : Sum
  Sum1 : Sum
  alpha0 : Constant  Value=disc.alpha0
  Cd : Outport
  wires:
  Sum1/1 -> Cd/1
  Square/1 -> Product/2
  Product/1 -> Sum1/2
  Cda/1 -> Product/1
  Cd0/1 -> Sum1/1
  Sum/1 -> Square/1
  alpha0/1 -> Sum/2
  alpha/1 -> Sum/1

== system flatball_6dof-old/lab/wrk/hummel/aero-coeff/Subsystem1 ==
  alpha : Inport
  CL0 : Constant  Value=disc.CL0
  CLa : Constant  Value=disc.CLa
  Product : Product
  Sum1 : Sum
  Cl : Outport
  wires:
  alpha/1 -> Product/2
  CL0/1 -> Sum1/1
  CLa/1 -> Product/1
  Product/1 -> Sum1/2
  Sum1/1 -> Cl/1

== system flatball_6dof-old/lab/wrk/hummel/aero-coeff/Subsystem2 ==
  alpha : Inport
  CM0 : Constant  Value=disc.CM0
  CMa : Constant  Value=disc.CMa
  Product : Product
  Sum1 : Sum
  Cm : Outport
  wires:
  Sum1/1 -> Cm/1
  Product/1 -> Sum1/2
  CMa/1 -> Product/1
  CM0/1 -> Sum1/1
  alpha/1 -> Product/2

== matlab function flatball_6dof-old/lab/helpers/Subsystem2/angle-of-attack ==
  data: Xdot input; alpha output
function alpha  = f( Xdot)
% calculate angle of attack

alpha = atan( Xdot(3) / Xdot(1));

== matlab function flatball_6dof-old/calc-Xdot ==
  data: X input; F input; Xdot output; Flaunch input
function Xdot   = f_lin( X, F, Flaunch)
% flatball equations of motion - NED (north-east-down) configuration
%

%% internal states
% x = X(1); y = X(2); z = X(3);
xdot = X(4); ydot = X(5); zdot = X(6);

Xdot = zeros(1,6);

%% define non-aerodynamic parameters
disc = struct;
disc.m = 0.175; % Kg


%%
xdotdot = (F(1) + Flaunch(1)) / disc.m;
ydotdot = (F(2) + Flaunch(2)) / disc.m;
zdotdot = (F(3) + Flaunch(3)) / disc.m;

%%
Xdot(1) = xdot;
Xdot(2) = ydot;
Xdot(3) = zdot;

Xdot(4) = xdotdot;
Xdot(5) = ydotdot;
Xdot(6) = zdotdot;

== matlab function flatball_6dof-old/lab/wrk/hummel/vector-norm ==
  data: vec input; norm output
function norm = fcn( vec)

norm = sqrt( vec(1)*vec(1) + vec(2)*vec(2) + vec(3)*vec(3));

== matlab function flatball_6dof-old/lab/wrk/hummel/Subsystem/Tc ==
  data: phi input; theta input; Tc output
function Tc = fcn( phi, theta)

sin_theta = sin( theta);
cos_theta = cos( theta);
sin_phi = sin( phi);
cos_phi = cos(phi);

Tc = [
    cos_theta sin_theta*sin_phi -sin_theta*cos_phi;
    0 cos_phi sin_phi;
    sin_theta -cos_theta*sin_phi cos_theta*cos_phi;
    ];

== matlab function flatball_6dof-old/lab/wrk/hummel/vp ==
  data: vel input; vp output; Tc input; vc3 input
function vp = fcn( vel, Tc, vc3)

c3 = Tc(:,3);

vp = [ vel - vc3*c3];

== matlab function flatball_6dof-old/lab/wrk/hummel/alpha ==
  data: v_N input; vc3 input; alpha output
function alpha = fcn( v_N, vc3)

alpha = atan( vc3 / norm( v_N)); % angle of attack

== matlab function flatball_6dof-old/lab/wrk/hummel/vc3 ==
  data: vel input; vc3 output; Tc input
function vc3 = fcn( vel, Tc)

c3 = Tc(:,3);
vc3 = dot( vel, c3);

== matlab function flatball_6dof-old/lab/wrk/c&p/Ta ==
  data: beta input; T output
function T  = Ta23( beta)
% transformation matrix
%

cos_beta = cos( beta);
sin_beta = sin( beta);

T = [ ...
    cos_beta -sin_beta 0;
    -sin_beta cos_beta 0;
    0 0 1;
    ];

== matlab function flatball_6dof-old/lab/wrk/hummel/F,M/vector-norm ==
  data: vec input; norm output
function norm = fcn( vec)

norm = sqrt( vec(1)*vec(1) + vec(2)*vec(2) + vec(3)*vec(3));

== matlab function flatball_6dof-old/lab/wrk/hummel/F,M/c3 ==
  data: Tc input; c3 output
function c3 = fcn( Tc)

c3 = Tc(:,3);

== matlab function flatball_6dof-old/lab/wrk/hummel/wD ==
  data: TH input; TH_dt input; wD output; Tc input
function wD = fcn( TH, TH_dt, Tc)

cos_theta = cos( TH(2));
sin_theta = sin( TH(2));

phidot = TH_dt(1);
thetadot = TH_dt(2);
gammadot = TH_dt(3);

wD_N_inC = [phidot*cos_theta thetadot phidot*sin_theta+gammadot];
wD = Tc' * wD_N_inC';

== matlab function flatball_6dof-old/lab/wrk/c&p/q-inf/vector-norm ==
  data: vec input; norm output
function norm = fcn( vec)

norm = sqrt( vec(1)*vec(1) + vec(2)*vec(2) + vec(3)*vec(3));

== matlab function flatball_6dof-old/lab/wrk/c&p/Subsystem1/transformation-matrices/Ta ==
  data: TH input; Ta12 output
function Ta12  = Ta( TH)
% transformation matrix
%
phi = TH(1); theta = TH(2); psi = TH(3);

cos_phi = cos( phi);
cos_theta = cos( theta);
cos_psi = cos( psi);

sin_phi = sin( phi);
sin_theta = sin( theta);
sin_psi = sin( psi);

Ta12 = [ ...
    cos_theta*cos_psi sin_phi*sin_theta*cos_phi-cos_phi*sin_psi cos_phi*sin_theta*cos_psi+sin_phi*sin_psi;
    cos_theta*sin_psi sin_phi*sin_theta*sin_psi+cos_phi*cos_psi cos_phi*sin_theta*sin_psi-sin_phi*cos_psi;
    -sin_theta sin_phi*cos_theta cos_phi*cos_theta
    ];

% cos_neg_phi = cos( -phi);
% cos_neg_theta = cos( -theta);
% cos_neg_psi = cos( -psi);
% 
% sin_neg_phi = sin( -phi);
% sin_neg_theta = sin( -theta);
% sin_neg_psi = sin( -psi);
% 
% Ta12 = [ ...
%     cos_neg_theta*cos_neg_psi sin_neg_phi*sin_neg_theta*cos_neg_phi-cos_neg_phi*sin_neg_psi cos_neg_phi*sin_neg_theta*cos_neg_psi+sin_neg_phi*sin_neg_psi;
%     cos_neg_theta*sin_neg_psi sin_neg_phi*sin_neg_theta*sin_neg_psi+cos_neg_phi*cos_neg_psi cos_neg_phi*sin_neg_theta*sin_neg_psi-sin_neg_phi*cos_neg_psi;
%     -sin_neg_theta sin_neg_phi*cos_neg_theta cos_neg_phi*cos_neg_theta
%     ];

== matlab function flatball_6dof-old/lab/wrk/c&p/Subsystem1/transformation-matrices/Tr ==
  data: TH input; Tr12 output
function Tr12  = Tr( TH)
% transformation matrix
%
phi = TH(1); theta = TH(2); psi = TH(3);

cos_phi = cos( phi);
cos_theta = cos( theta);
cos_psi = cos( psi);

sin_phi = sin( phi);
sin_theta = sin( theta);
sin_psi = sin( psi);

Tr12 = [
    1 0 -sin_theta;
    0 cos_phi cos_theta*sin_psi;
    0 -sin_phi cos_theta*cos_psi;
    ];

== matlab function flatball_6dof-old/lab/wrk/c&p/Subsystem1/w_ ==
  data: THdot input; M output
function M  = w_( THdot)
% transformation matrix
%
p = THdot(1); q = THdot(2); r = THdot(3);

M = [ ...
    0 -r q;
    r 0 -p;
    -q p 0
    ];

== matlab function flatball_6dof-old/lab/wrk/c&p/Ta1 ==
  data: alpha input; T output
function T  = Ta34( alpha)
% transformation matrix
%

cos_alpha = cos( alpha);
sin_alpha = sin( alpha);

T= [ ...
    cos_alpha 0 -sin_alpha;
    0 1 0;
    sin_alpha 0 cos_alpha;
    ];

== matlab function flatball_6dof-old/lab/wrk/c&p/angle-of-attack ==
  data: Xdot input; alpha output
function alpha  = f( Xdot)
% calculate angle of attack

alpha = atan2( Xdot(3) / Xdot(1));

== matlab function flatball_6dof-old/lab/wrk/c&p/zero-side-slip-angle ==
  data: Xdot input; beta output
function beta  = f( Xdot)
% calculate side-slip angle

y = Xdot(2);
x = Xdot(1);

beta = atan2( y / x);

== matlab function flatball_6dof-old/lab/wrk/flatball_6dof_v1p1 ==
  data: X input; Xdot output; lift output; drag output; alpha output; AdvR output; E_trans output; E_rot output
function [Xdot, lift, drag, alpha, AdvR, E_trans, E_rot]  = flatball_6dof_eom( X)
% flatball equations of motion - NED (north-east-down) configuration
%

%% internal states
x = X(1); y = X(2); z = X(3);
xdot = X(4); ydot = X(5); zdot = X(6);

phi = X(7); theta = X(8); gamma = X(9);
phidot = X(10); thetadot = X(11); gammadot = X(12);

Xdot = zeros(1,12);

%% define ambient parameters
amb.g = 9.81; % m/s^2
amb.rho = 1.23; % Kg/m^3

%% define non-aerodynamic parameters
disc = struct;
disc.m = 0.175; % Kg
disc.A = 0.057; % m^2
disc.d = 2*sqrt(0.057/pi); % 2*sqrt(disc.A/pi); % diameter
disc.Ia = 0.002352; % moment of inertia about the spinning axis
disc.Id = 0.001219; % moment of inertia about the planar axis'

%% crowther and potts - per hummel and hubbard
% disc.CL0 = 0.13;
% disc.CLa = 3.09;
% disc.CD0 = 0.085;
% disc.CDa = 3.30;
% disc.CM0 = -0.01;
% disc.CMa = 0.057;
% 
% disc.CMq = 0.0008; % NOTE: not used
% disc.CLr = 0.0004;
% disc.CLp = -0.013;
% disc.CNr = -2.8e-5;
% 
% disc.alpha0 = -0.052; % rad

%% hummel and hubbard 2014
disc.CL0 = 0.188;
disc.CLa = 2.37;

disc.CD0 = 0.15;
disc.CDa = 1.24;

disc.CM0 = -0.06;
disc.CMa = 0.38;

disc.CMq = 0.0008; % NOTE: not used
disc.CLr = 0.0004;

disc.CNr = -2.8e-5;

disc.CLp = -0.013;

% disc.CRr = 1.4e-2; % NOTE: missing from 2014, borrowed from 2003 thesis
% disc.CRr = 3e-3; % NOTE: missing from 2014, borrowed from P&C
disc.CRr = 0.00171; % appendix of hummel thesis
disc.CRp =-5.5e-3; % NOTE: missing from 2014, borrowed from P&C

% not sure where these are from...
% disc.CMq= -1.44E-02;
% disc.CRp =-1.25E-02;
% disc.CNr = -3.41E-05; % long flight f2302

disc.alpha0 = -0.052; % rad

%% helper variables
sin_theta = sin( theta);
cos_theta = cos( theta);
sin_phi = sin( phi);
cos_phi = cos(phi);

% c = T_c_N * N --> transformation matrix T_c_N in N reference frame
T_c_N = [cos_theta sin_theta*sin_phi -sin_theta*cos_phi;
    0 cos_phi sin_phi;
    sin_theta -cos_theta*sin_phi cos_theta*cos_phi];
% c1 = T_c_N(1,:);
% c2 = T_c_N(2,:);
c3 = T_c_N(3,:);

%% aerodynamic forces and moments in N reference frame
vel = [xdot ydot zdot];
vmag = norm( vel);
vc3 = dot( vel, c3);
v_N = [ vel - vc3*c3];
Adp = 0.5 * disc.A * amb.rho * vmag*vmag;
uvel = vel / vmag;
uv_N = v_N / norm( v_N);
u_lat = cross( c3, uv_N);

wD_N_inC = [phidot*cos_theta thetadot phidot*sin_theta+gammadot];
wD_N_inN = T_c_N' * wD_N_inC';

w_v_N = dot( wD_N_inN, uv_N);
w_lat = dot( wD_N_inN, u_lat);
w_spin = dot( wD_N_inN, c3);

alpha = atan( vc3 / norm( v_N)); % angle of attack
AdvR = disc.d * w_spin / 2 / vmag; % advance ratio
E_trans = 0.5 * disc.m * vmag*vmag; % translational energy
E_rot = 0.5 * disc.Ia * gammadot*gammadot; % rotational energy

%% hacks
k_spin_down_decay = 0.25;
% k_CL_gain = 1.0; %2.5;
% k_CD_gain = 1.0; %1.5;
% k_M_gain = 1.0;

%% coefficients - f(alpha)
dalpha = alpha - disc.alpha0;
CL = disc.CL0 + disc.CLa * alpha;
CD = disc.CD0 + disc.CDa * dalpha*dalpha;
CM = disc.CM0 + disc.CMa * alpha;
Mv_N = Adp * disc.d * (sqrt(disc.d/amb.g)*disc.CRr*w_spin + disc.CRp*w_v_N) * uv_N;

%% coefficients - lookup based
% 
% CL = interp1( disc.CL_data(:,1), disc.CL_data(:,2).*k_CL_gain, alpha, 'spline');
% CD = interp1( disc.CD_data(:,1), disc.CD_data(:,2).*k_CD_gain, alpha, 'spline');
% CM = interp1( disc.CM_data(:,1), disc.CM_data(:,2).*k_M_gain, alpha, 'spline');
% % CRr = interp2( disc.CRr_rad, disc.CRr_AdvR, disc.CRr_data, alpha, AdvR,'spline');
% Mv_N = Adp * disc.d * ( disc.CRr* + disc.CRp*w_v_N) * uv_N;

%%
lift = CL * Adp;
drag = CD * Adp;
ulift = -cross( uvel, u_lat);
udrag = -uvel;
Faero = lift*ulift + drag*udrag;
Fg_N = [0 0 disc.m*amb.g]';

F = Faero' + Fg_N;

Mlat = Adp * disc.d * (CM + disc.CMq * w_lat) * u_lat;
Mspin = [0 0 disc.CNr*w_spin];
M = T_c_N * Mv_N' + T_c_N*Mlat' + Mspin';

%%
xdotdot = F(1) / disc.m;
ydotdot = F(2) / disc.m;
zdotdot = F(3) / disc.m;

phidotdot = (M(1) + disc.Id*thetadot*phidot*sin_theta - disc.Ia*thetadot*(phidot*sin_theta+gammadot) + disc.Id*thetadot*phidot*sin_theta)/disc.Id/cos_theta; 
thetadotdot = (M(2) + disc.Ia*phidot*cos_theta*(phidot*sin_theta +gammadot) - disc.Id*phidot*phidot*cos_theta*sin_theta)/disc.Id;
gammadotdot = (M(3) - disc.Ia*(k_spin_down_decay*gammadot*sin_theta + thetadot*phidot*cos_theta))/disc.Ia;

% bug in hummels report?
% gammadotdot = (M(3) - disc.Ia*(phidotdot*sin_theta + thetadot*phidot*cos_theta))/disc.Ia;
% bug in hummels report?
% w/phidotdot term, there is no decay in gammadot
% w/out gammadot term - there is no decay in gammadot
% NOTE: w/it, the decay is too agressive
% FIXME: investigate why this term is necessary for more appropriate
% spindown (based on my data)

%%
Xdot(1) = xdot;
Xdot(2) = ydot;
Xdot(3) = zdot;

Xdot(4) = xdotdot;
Xdot(5) = ydotdot;
Xdot(6) = zdotdot;

Xdot(7) = phidot;
Xdot(8) = thetadot;
Xdot(9) = gammadot;

Xdot(10) = phidotdot;
Xdot(11) = thetadotdot;
Xdot(12) = gammadotdot;

== matlab function flatball_6dof-old/lab/rotations/X-to-T_c_N ==
  data: X input; T_c_N output
function T_c_N  = f( X)
%% internal states
phi = X(7); theta = X(8);

%% helper variables
sin_theta = sin( theta);
cos_theta = cos( theta);
sin_phi = sin( phi);
cos_phi = cos(phi);

T_c_N = [
    cos_theta sin_theta*sin_phi -sin_theta*cos_phi;
    0 cos_phi sin_phi;
    sin_theta -cos_theta*sin_phi cos_theta*cos_phi
    ];

== matlab function flatball_6dof-old/lab/alpha- ==
  data: X input; alpha output; T_c_N input
function alpha  = f( X, T_c_N)
%% internal states
xdot = X(4); ydot = X(5); zdot = X(6);

%% helper variables
T_c_Npsi = T_c_N(3,:);

vel = [xdot ydot zdot];
vc3 = dot( vel, T_c_Npsi);
v_N = [ vel - vc3*T_c_Npsi];

alpha = atan( vc3 / norm( v_N)); % angle of attack

== matlab function flatball_6dof-old/lab/rotations/X-to-wD_N_inC ==
  data: X input; wD_N_inC output
function wD_N_inC  = f( X)
%% internal states
theta = X(8);
phidot = X(10); thetadot = X(11); gammadot = X(12);

%% helper variables
sin_theta = sin( theta);
cos_theta = cos( theta);

wD_N_inC = [phidot*cos_theta thetadot phidot*sin_theta+gammadot];

== matlab function flatball_6dof-old/lab/calc-F/q-inf/vector-norm ==
  data: vec input; norm output
function norm = fcn( vec)

norm = sqrt( vec(1)*vec(1) + vec(2)*vec(2) + vec(3)*vec(3));

== matlab function flatball_6dof-old/lab/calc-F/q-inf/X-to-vel ==
  data: X input; vel output
function vel = fcn( X)
xdot = X(4); ydot = X(5); zdot = X(6);
vel = [xdot ydot zdot];

== matlab function flatball_6dof-old/lab/calc-F/X-to-vel ==
  data: X input; vel output
function vel = fcn( X)
xdot = X(4); ydot = X(5); zdot = X(6);
vel = [xdot ydot zdot];
